simulink model "Biglide_Lee_Palma"  (R2019b)
settings: Solver=VariableStepAuto  StartTime=0.0  StopTime=3  RelTol=1e-3
values from neighbouring files (symbols this model uses):
  ADAMS_communication_interval = 0.005    [Controls_Plant_1.m]    (also in Controls_Plant_3.m; Controls_Plant_5.m)
  ADAMS_communications_per_output_step = 1    [Controls_Plant_1.m]    (also in Controls_Plant_3.m; Controls_Plant_5.m)
  ADAMS_cwd = 'C:\Users\Justin\Documents\EMARO+\Centrale Nantes\Courses\AMORO\Lab\Lab 4'    [Controls_Plant_1.m]    (also in Controls_Plant_3.m; Controls_Plant_5.m)
  ADAMS_exec = ''    [Controls_Plant_1.m]    (also in Controls_Plant_3.m; Controls_Plant_5.m)
  ADAMS_host = 'LAPTOP-CH4PO0JS'    [Controls_Plant_1.m]    (also in Controls_Plant_3.m; Controls_Plant_5.m)
  ADAMS_init = ''    [Controls_Plant_1.m]    (also in Controls_Plant_3.m; Controls_Plant_5.m)
  ADAMS_inputs = 'dummy_input'    [Controls_Plant_1.m]    (also in Controls_Plant_3.m = 'q1d!q2d'; Controls_Plant_5.m = 'f1!f2')
  ADAMS_outputs = 'x!y!xd!yd!xdd!ydd!phi1!phi2!phi1d!phi2d!phi1dd!phi2dd!f1!f2'    [Controls_Plant_1.m]    (also in Controls_Plant_3.m = 'q1!q2'; Controls_Plant_5.m = 'q1!q2')
  ADAMS_prefix = 'Controls_Plant_1'    [Controls_Plant_1.m]    (also in Controls_Plant_3.m = 'Controls_Plant_3'; Controls_Plant_5.m = 'Controls_Plant_5')
  ADAMS_static = 'no'    [Controls_Plant_1.m]    (also in Controls_Plant_3.m; Controls_Plant_5.m)
  ADAMS_sysdir = 'C:\PROGRA~1\MSC~1.SOF\ADAMSS~1\2020_1\'    [Controls_Plant_1.m]    (also in Controls_Plant_3.m; Controls_Plant_5.m)
  ADAMS_time_offset = 0.0    (= 0)    [Controls_Plant_1.m]    (also in Controls_Plant_3.m; Controls_Plant_5.m)
settings Model: Creator=Steven  LastModifiedBy=Justin
settings DataIOCC: ReturnWorkspaceOutputs=off
settings DebuggingCC: ArithmeticOperatorsInVariantConditions=warning
settings SFSimCC: SimUseLocalCustomCode=off  CustomCodeUndefinedFunction=UseInterfaceOnly
settings RTWCC: RTWUseLocalCustomCode=off

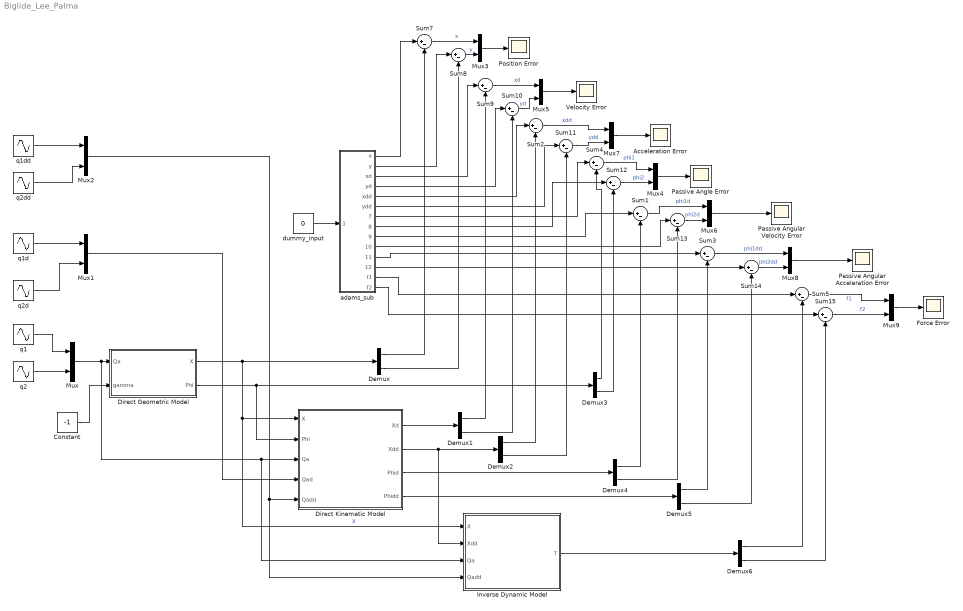
== system Biglide_Lee_Palma ==
  Acceleration Error : Scope
  Constant : Constant  Value=-1
  Demux{,1..6} (7 alike) : Demux  Outputs=2
  Direct Geometric Model : MATLAB Function  TreatAsAtomicUnit=on
  Direct Kinematic Model : MATLAB Function  TreatAsAtomicUnit=on
  Force Error : Scope
  Inverse Dynamic Model : MATLAB Function  TreatAsAtomicUnit=on
  Mux{,1..9} (10 alike) : Mux  Inputs=2
  Passive Angle Error : Scope
  Passive Angular Acceleration Error : Scope
  Passive Angular Velocity Error : Scope
  Position Error : Scope
  Sum{1..5,7..15} (14 alike) : Sum  Inputs=|+-
  Velocity Error : Scope
  adams_sub : Subsystem
  dummy_input : Constant  Value=0
  q1 : Sin  Amplitude=0.1  SampleTime=0
  q1d : Sin  Amplitude=0.1  Phase=+pi/2  SampleTime=0
  q1dd : Sin  Amplitude=0.1  Phase=+pi  SampleTime=0
  q2 : Sin  Amplitude=-0.1  SampleTime=0
  q2d : Sin  Amplitude=-0.1  Phase=pi/2  SampleTime=0
  q2dd : Sin  Amplitude=-0.1  Phase=+pi  SampleTime=0
  wires:
  q1/1 -> Mux/1
  q2/1 -> Mux/2
  Mux/1 -> Inverse Dynamic Model/3(Qa), Direct Kinematic Model/3(Qa), Direct Geometric Model/1(Qa)
  Constant/1 -> Direct Geometric Model/2(gamma)
  Direct Geometric Model/2(Phi) -> Direct Kinematic Model/2(Phi), Demux3/1
  q1d/1 -> Mux1/1
  q2d/1 -> Mux1/2
  Mux1/1 -> Direct Kinematic Model/4(Qad)
  q1dd/1 -> Mux2/1
  q2dd/1 -> Mux2/2
  Mux2/1 -> Inverse Dynamic Model/4(Qadd), Direct Kinematic Model/5(Qadd)
  Direct Kinematic Model/1(Xd) -> Demux1/1
  Direct Kinematic Model/2(Xdd) -> Demux2/1, Inverse Dynamic Model/2(Xdd)
  Direct Kinematic Model/3(Phid) -> Demux4/1
  Direct Kinematic Model/4(Phidd) -> Demux5/1
  adams_sub/14("f2    ") -> Sum15/1
  adams_sub/13("f1    ") -> Sum5/1
  adams_sub/12(phi2dd) -> Sum14/1
  adams_sub/11(phi1dd) -> Sum3/1
  adams_sub/10("phi2d ") -> Sum13/1
  adams_sub/9("phi1d ") -> Sum1/1
  adams_sub/8("phi2  ") -> Sum12/1
  adams_sub/7("phi1  ") -> Sum4/1
  adams_sub/6("ydd   ") -> Sum11/1
  adams_sub/5("xdd   ") -> Sum2/1
  adams_sub/4("yd    ") -> Sum10/1
  adams_sub/3("xd    ") -> Sum9/1
  adams_sub/2("y     ") -> Sum8/1
  adams_sub/1("x     ") -> Sum7/1
  dummy_input/1 -> adams_sub/1(dummy_input)
  Mux3/1 -> Position Error/1
  Mux4/1 -> Passive Angle Error/1
  Mux5/1 -> Velocity Error/1
  Mux7/1 -> Acceleration Error/1
  Mux8/1 -> Passive Angular Acceleration Error/1
  Mux9/1 -> Force Error/1
  Direct Geometric Model/1(X) -> Inverse Dynamic Model/1(X), Direct Kinematic Model/1(X), Demux/1  "X"
  Sum7/1 -> Mux3/1  "x"
  Demux/1 -> Sum7/2
  Demux/2 -> Sum8/2
  Sum8/1 -> Mux3/2  "y"
  Demux1/1 -> Sum9/2
  Demux1/2 -> Sum10/2
  Sum9/1 -> Mux5/1  "xd"
  Sum10/1 -> Mux5/2  "yd"
  Demux2/1 -> Sum2/2
  Demux2/2 -> Sum11/2
  Sum2/1 -> Mux7/1  "xdd"
  Sum11/1 -> Mux7/2  "ydd"
  Sum12/1 -> Mux4/2  "phi2"
  Sum4/1 -> Mux4/1  "phi1"
  Demux3/1 -> Sum4/2
  Demux3/2 -> Sum12/2
  Sum1/1 -> Mux6/1  "phi1d"
  Sum13/1 -> Mux6/2  "phi2d"
  Demux4/1 -> Sum1/2
  Demux4/2 -> Sum13/2
  Mux6/1 -> Passive Angular Velocity Error/1
  Sum14/1 -> Mux8/2  "phi2dd"
  Sum3/1 -> Mux8/1  "phi1dd"
  Demux5/1 -> Sum3/2
  Demux5/2 -> Sum14/2
  Inverse Dynamic Model/1(T) -> Demux6/1
  Sum5/1 -> Mux9/1  "f1"
  Sum15/1 -> Mux9/2  "f2"
  Demux6/1 -> Sum5/2
  Demux6/2 -> Sum15/2

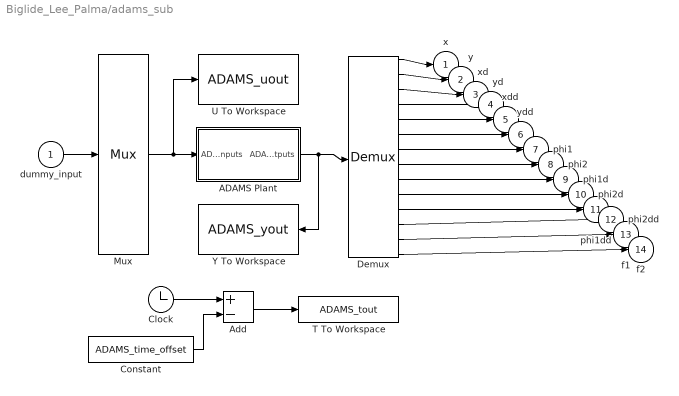
== system Biglide_Lee_Palma/adams_sub ==
  dummy_input : Inport
  ADAMS Plant : Subsystem  LoadFcn=|  InitFcn=clear mex  mask(Adams Plant){exevie=ADAMS_sysdir, nam_in=ADAMS_inputs, namout=ADAMS_outputs, nampre=ADAMS_prefix, outfil=ADAMS_prefix, exesol=ADAMS_exec, stat=ADAMS_static, inicmd=[ADAMS_init], exetyp=C++, comtyp=PIPE(DDE), workdir=ADAMS_cwd, ada_host=ADAMS_host, modani=interactive, modsim=discrete, dft=no, simulink_lead_cosim=yes, pin_interp_order=0, pout_extrap_order=0, pin_extrap_order=0, pout_interp_order=0, dt_out=ADAMS_communication_interval, o_rate=ADAMS_communications_per_output_step, time_offset=ADAMS_time_offset, more=off}
      | %check based on dialog box setting for when setting by popup menu                                             
      | if exist('ADAMS_solver_type')                                                                                 
      |   if strcmp(ADAMS_solver_type,'C++')                                                                          
      |     set_param(gcb,'exetyp','C++');                                                                            
      |   else                                                                                                        
      |     set_param(gcb,'exetyp','Fortran');                                                                        
      |   end                                                                                                         
      | else                                                                                                          
      |   set_param(gcb,'exetyp','C++');                                                                              
      | end                                                                                                           
      | %set the mode if using acar_solver                                                                            
      | %REQUIRED HERE BECAUSE BELOW CAUSES MDLTERMINATE TO BE CALLED 2 TIMES IN MIDDLE OF SIMULATION WHEN SET IN MASK
      |                                                                                                               
      | %enable the direct feedthrough, sim mode, anim mode parameters by default                                     
      |                                                                                                               
      | if exist('set_some_params_states')                                                                            
      |                                                                                                               
      |   set_some_params_states({'dft','modsim','modani'},{'on','on','on'},'MaskEnables',gcb)                        
      |   %turn on direct feedthrough option                                                                          
      |   set_some_params_states({'dft'},{'on'},'MaskVisibilities',gcb)                                               
      |                                                                                                               
      |  end                                                                                                          
      |                                                                                                               
      |                                                                                                               
      | if exist('ADAMS_exec')                                                                                        
      |   if and(strcmp(get_param(gcb,'exesol'),'ADAMS_exec'),strcmp(ADAMS_exec,'acar_solver'))                       
      |     %set the sim mode to discrete -- only supported mode                                                      
      |     set_param(gcb,'modsim','discrete')                                                                        
      |      %turn off direct feedthrough option                                                                      
      |      set_some_params_states({'dft'},{'off'},'MaskVisibilities',gcb)                                           
      |     %set the animation mode to batch -- only supported mode                                                   
      |     set_param(gcb,'modani','batch')                                                                           
      |     %disable the direct feedthrough, sim mode, anim mode parameters                                           
      |     set_some_params_states({'modsim','modani'},{'off','off'},'MaskEnables',gcb)                               
      |   end
      |   if and(strcmp(get_param(gcb,'exesol'),'ADAMS_exec'),strcmp(ADAMS_exec,'apre_solver'))                       
      |     %set the sim mode to discrete -- only supported mode                                                      
      |     set_param(gcb,'modsim','discrete')                                                                        
      |      %turn off direct feedthrough option                                                                      
      |      set_some_params_states({'dft'},{'off'},'MaskVisibilities',gcb)                                           
      |     %set the animation mode to batch -- only supported mode                                                   
      |     set_param(gcb,'modani','batch')                                                                           
      |     %disable the direct feedthrough, sim mode, anim mode parameters                                           
      |     set_some_params_states({'modsim','modani'},{'off','off'},'MaskEnables',gcb)                               
      |   end                                                                                                  
      | end
      mask prompts: exevie "Adams install directory"; nam_in "Adams View input names"; namout "Adams View output names"; nampre "Adams model file prefix"; outfil "Output files prefix (opt.: if blank - no output)"; exesol "User executable (opt.: if blank - use standard)"; stat "Initial static simulation flag"; inicmd "Initialization commands"; exetyp "Adams Solver type"; comtyp "Interprocess option"; workdir "Adams working directory"; ada_host "Adams host"; modani "Animation mode"; modsim "Simulation mode"; dft "Direct feedthrough"; simulink_lead_cosim "Discrete Computational Order - Simulink Leads Adams"; pin_interp_order "Plant input interpolation order"; pout_extrap_order "Plant output extrapolation order"; pin_extrap_order "Plant input extrapolation order"; pout_interp_order "Plant output interpolation order"; dt_out "Communication interval"; o_rate "Number of communications per output step"; time_offset "Offset between Simulink and Adams simulation time"; more "More parameters"
      mask help: Simulate any Adams plant model either in Adams Solver form (.adm file) or in Adams View form (.cmd file)
      settings: OpenFcn=|
      | open_system(gcb,'mask')
      | if not(exist('set_some_params_states'))
      | 
      | warning('The script "set_some_params_states.m" cannot be found in the MATLAB PATH.  Cannot update the ADAMS Plant S-Function parameters.')
      | 
      | warning('Recommended action(optional):  run the Adams Controls .m file first to help choose the correct settings in the Adams S-Function block.')
      | 
      | end
      mask Help:
      | <html>
      | This S-Function represents the non-linear Adams Plant with the inputs sent to the Adams model as input #1 and Time as input #2<br>
      |  and the outputs generated by the Adams model.  See the Adams Controls documentation for more <br>
      | information.  This plant uses the following variables:<br>
      | <br>
      | <b>ADAMS_sysdir:</b> Adams installation directory<br>
      | <b>ADAMS_inputs:</b> Input variables View names vector<br>
      | <b>ADAMS_outputs :</b> Outputs variables View names vector<br>
      | <b>ADAMS_prefix:</b> ADAMS model files prefix (.adm, .cmd); also doubles as output files prefix<br>
      | <b>ADAMS_exec:</b>  Adams Solver user library or keyword (e.g., acar_solver)<br>
      | <b>ADAMS_static:</b> yes|no - initial static before Co-simulation(discrete)/Function Evaluation(continuous)<br>
      | <b>ADAMS_init:</b> Initialization commands (i.e., Adams View or Solver commands, depending on setting for Animation mode)<br>
      | <b>ADAMS_cwd:</b> Current working directory (for TCP/IP)<br>
      | <b>ADAMS_host:</b> Name of Adams server host (for TCP/IP)<br>
      | <b>ADAMS_mode:</b> Linear or non-linear (i.e., co-sim, function eval)<br>
      | <b>ADAMS_solver_type:</b> Fortran or C++ (used to set popup menu when first loaded)<br>
      | <b>ADAMS_communication_interval:</b> Time step at which Co-simulation exchange information (e.g.,0.005); also controls <br>output for continuous mode (Function Evaluation)<br>
      | <b>ADAMS_communications_per_output_step: </b>Sets Adams output rate (.res, .req, .gra) integer value (default: 1)<br>
      | <b>ADAMS_time_offset: </b>Removes this time offset from simulation time used by Adams. Adams will be sent a time value being Simulink simulation time - this value. (default: 0). Eg. if ADAMS_time_offset=2: if Simulink time=2 then Adams time = 0. Make sure that the Adams block is disabled when the Adams time is <0. If not an error will be raised. <br>
      | 
      | 
      | <br>
      | The following settings can be chosen:<br>
      | <br>
      | <b>Adams Solver type:</b>  Fortran or C++ (will also set ADAMS_solver_type)<br>
      | <b>Interprocess option:</b> Pipe(DDE), TCP/IP or DIRECT; TCP/IP can allow different machines run Adams and MATLAB<br>
      | <b>Animation mode:</b> batch (Solver, uses .adm) or interactive (View, uses .cmd)<br>
      | <b>Simulation mode:</b> discrete (Co-simulation) or continuous (Function Evaluation)<br>
      | <b>Discrete Computational Order - Simulink Lead Adams:</b> for discrete mode, chooses if Simulink leads the integration (yes) or lags (no);<br> if set to "no", can remove algebraic loop<br>
      | <b>Plant input interpolation order:</b> 0 = zero-order hold; 1 = linear (discrete mode only, where Simulink leads)<br>
      | <b>Plant output extrapolation order:</b> 0 = zero-order hold;1 = linear(discrete mode only, where Simulink leads)<br>
      | <b>Plant input extrapolation order:</b> 0 = zero-order hold; 1 = linear (discrete mode only, where Adams leads)<br>
      | <b>Plant output interpolation order:</b> 0 = zero-order hold;1 = linear(discrete mode only, where Adams leads)<br>
      | <b>Direct feedthrough:</b> yes|no - yes = Input directly effect output(continuous mode-only)<br>
      | 
      | </html>
      mask Callback exesol:
      | if exist('set_some_params_states')
      | %enable the direct feedthrough, sim mode, anim mode parameters
      | set_some_params_states({'dft','modsim','modani'},{'on','on','on'},'MaskEnables',gcb)
      | %turn on direct feedthrough option
      | set_some_params_states({'dft'},{'on'},'MaskVisibilities',gcb)
      | end
      | 
      | if exist('ADAMS_exec')
      |   if and(strcmp(get_param(gcb,'exesol'),'ADAMS_exec'),strcmp(ADAMS_exec,'acar_solver'))
      |     %set the sim mode to discrete -- only supported mode
      |     %REMOVED:  BELOW CAUSES MDLTERMINATE TO BE CALLED 2 TIMES IN MIDDLE OF SIMULATION
      |     %Now in LoadFcn callback
      |     %set_param(gcb,'modsim','discrete')
      |      %turn off direct feedthrough option
      |     set_some_params_states({'dft'},{'off'},'MaskVisibilities',gcb)
      |     %set the animation mode to batch -- only supported mode
      |     %REMOVED:  BELOW CAUSES MDLTERMINATE TO BE CALLED 2 TIMES IN MIDDLE OF SIMULATION
      |     %Now in LoadFcn callback
      |     %set_param(gcb,'modani','batch')
      |     %disable the direct feedthrough, sim mode, anim mode parameters
      |     set_some_params_states({'modsim','modani'},{'off','off'},'MaskEnables',gcb)
      |   end
      | end
      mask TypeOptions exetyp: Fortran | C++
      mask Callback exetyp:
      | if strcmp(get_param(gcb,'exetyp'),'C++')
      |     ADAMS_solver_type='C++';
      | else
      |     ADAMS_solver_type='Fortran';
      | end
      mask TypeOptions comtyp: PIPE(DDE) | TCP/IP | DIRECT
      mask Callback comtyp:
      | if exist('set_some_params_states')
      | if strcmp(get_param(gcb,'comtyp'),'PIPE(DDE)') || strcmp(get_param(gcb,'comtyp'),'DIRECT')
      |     %turn off cwd, host options
      |     set_some_params_states({'ada_host','workdir'},{'off','off'},'MaskVisibilities',gcb)
      | else%if strcmp(get_param(gcb,'modsim'),'TCP/IP')
      |     %turn on cwd, host options
      |     set_some_params_states({'ada_host','workdir'},{'on','on'},'MaskVisibilities',gcb)
      | end
      | end
      mask TypeOptions modani: batch | interactive
      mask TypeOptions modsim: discrete | continuous
      mask Callback modsim:
      | if exist('set_some_params_states')
      | if strcmp(get_param(gcb,'modsim'),'discrete')
      |      %turn off direct feedthrough option
      |     set_some_params_states({'dft'},{'off'},'MaskVisibilities',gcb)
      |     %turn on discrete co-sim type if want to see more
      |     if strcmp(get_param(gcb,'more'),'on')
      |         set_some_params_states({'simulink_lead_cosim'},{'on'},'MaskVisibilities',gcb)
      |     end
      |     if strcmp(get_param(gcb,'simulink_lead_cosim'),'yes')
      |         %turn on interpolation/extrapolation options
      |         set_some_params_states({'pin_interp_order','pout_extrap_order',},{'on','on'},'MaskVisibilities',gcb)
      |     else
      |         set_some_params_states({'pin_extrap_order','pout_interp_order'},{'on','on'},'MaskVisibilities',gcb)
      |     end
      | else%if strcmp(get_param(gcb,'modsim'),'continuous')
      |      %turn off direct feedthrough option
      |     set_some_params_states({'dft'},{'on'},'MaskVisibilities',gcb)
      |     %turn off interpolation/extrapolation options
      |     set_some_params_states({'pin_interp_order','pout_extrap_order','pin_extrap_order','pout_interp_order','simulink_lead_cosim'},{'off','off','off','off','off'},'MaskVisibilities',gcb)
      | end
      | end
      mask TypeOptions dft: no | yes
      mask TypeOptions simulink_lead_cosim: yes | no
      mask Callback simulink_lead_cosim:
      | if exist('set_some_params_states')
      | if (strcmp(get_param(gcb,'simulink_lead_cosim'),'yes') && strcmp(get_param(gcb,'modsim'),'discrete'))
      |      %turn off unused interpolate/extrapolate options
      |     set_some_params_states({'pin_extrap_order','pout_interp_order'},{'off','off'},'MaskVisibilities',gcb)
      |     %turn on used interpolate/extrapolate options
      |     set_some_params_states({'pin_interp_order','pout_extrap_order'},{'on','on'},'MaskVisibilities',gcb)
      | elseif (strcmp(get_param(gcb,'simulink_lead_cosim'),'no') && strcmp(get_param(gcb,'modsim'),'discrete'))
      |     %turn on used interpolate/extrapolate options
      |     set_some_params_states({'pin_extrap_order','pout_interp_order'},{'on','on'},'MaskVisibilities',gcb)
      |      %turn off unused interpolate/extrapolate options
      |     set_some_params_states({'pin_interp_order','pout_extrap_order'},{'off','off'},'MaskVisibilities',gcb)
      | end
      | end
      mask TypeOptions pin_interp_order: 0 | 1
      mask TypeOptions pout_extrap_order: 0 | 1
      mask TypeOptions pin_extrap_order: 0 | 1
      mask TypeOptions pout_interp_order: 0 | 1
      mask Callback more:
      | if exist('set_some_params_states')
      | if (strcmp(get_param(gcb,'more'),'on'))
      |      %turn on infrequently used options
      |     set_some_params_states({'exevie','nam_in','namout','exesol','stat','inicmd','time_offset'},{'on','on','on','on','on','on','on'},'MaskVisibilities',gcb)
      |     if strcmp(get_param(gcb,'modsim'),'discrete')
      |         set_some_params_states({'simulink_lead_cosim'},{'on'},'MaskVisibilities',gcb)
      |     end
      | elseif (strcmp(get_param(gcb,'more'),'off'))
      |     %turn off infrequently used options
      |     set_some_params_states({'exevie','nam_in','namout','exesol','stat','inicmd','time_offset'},{'off','off','off','off','off','off','off'},'MaskVisibilities',gcb)
      |     if strcmp(get_param(gcb,'modsim'),'discrete')
      |         set_some_params_states({'simulink_lead_cosim'},{'off'},'MaskVisibilities',gcb)
      |     end
      | end
      | end
      mask Display: disp( 'MSC Software' )
  Add : Sum  Inputs=+-
  Clock : Clock
  Constant : Constant  Value=ADAMS_time_offset
  Demux : Demux  Outputs=14
  Mux : Mux  Inputs=1
  T To Workspace : ToWorkspace  VariableName=ADAMS_tout
      settings: MaxDataPoints=100000
  U To Workspace : ToWorkspace  VariableName=ADAMS_uout
      settings: MaxDataPoints=100000
  Y To Workspace : ToWorkspace  VariableName=ADAMS_yout
      settings: MaxDataPoints=100000
  "x     " : Outport
  "y     " : Outport  Port=2
  "xd    " : Outport  Port=3
  "yd    " : Outport  Port=4
  "xdd   " : Outport  Port=5
  "ydd   " : Outport  Port=6
  "phi1  " : Outport  Port=7
  "phi2  " : Outport  Port=8
  "phi1d " : Outport  Port=9
  "phi2d " : Outport  Port=10
  phi1dd : Outport  Port=11
  phi2dd : Outport  Port=12
  "f1    " : Outport  Port=13
  "f2    " : Outport  Port=14
  wires:
  Mux/1 -> ADAMS Plant/1(ADAMS inputs), U To Workspace/1
  ADAMS Plant/1(ADAMS outputs) -> Demux/1, Y To Workspace/1
  Clock/1 -> Add/1
  Constant/1 -> Add/2
  Add/1 -> T To Workspace/1
  Demux/1 -> "x     "/1
  Demux/2 -> "y     "/1
  Demux/3 -> "xd    "/1
  Demux/4 -> "yd    "/1
  Demux/5 -> "xdd   "/1
  Demux/6 -> "ydd   "/1
  Demux/7 -> "phi1  "/1
  Demux/8 -> "phi2  "/1
  Demux/9 -> "phi1d "/1
  Demux/10 -> "phi2d "/1
  Demux/11 -> phi1dd/1
  Demux/12 -> phi2dd/1
  Demux/13 -> "f1    "/1
  Demux/14 -> "f2    "/1
  dummy_input/1 -> Mux/1

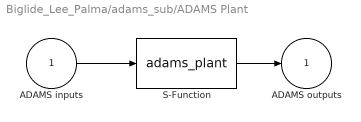
== system Biglide_Lee_Palma/adams_sub/ADAMS Plant ==
  ADAMS inputs : Inport
  S-Function : S-Function  StopFcn=clear mex  FunctionName=adams_plant  Parameters=exevie,exesol,stat,outfil,nampre,o_rate,nam_in,namout,dft,modsim,modani,dt_out,inicmd,exetyp,comtyp,ada_host, workdir,pin_interp_order,pout_extrap_order,pin_extrap_order,pout_interp_order,simulink_lead_cosim,time_offset  SFunctionDeploymentMode=off  EnableBusSupport=off
  ADAMS outputs : Outport  InitialOutput=0
  wires:
  ADAMS inputs/1 -> S-Function/1
  S-Function/1 -> ADAMS outputs/1

== matlab function Biglide_Lee_Palma/Direct Kinematic Model ==
  data: X input; Phi input; Xd output; Qa input; Qad input; Xdd output; Qadd input; Phid output; Phidd output
function [Xd, Xdd, Phid, Phidd]  = DKM(X,Phi,Qa,Qad,Qadd)
    
    %% Geometric parameters
    d= 0.4;
    l= 0.3606;
    
    % Extracting Parameters
    x = X(1);
    y = X(2);
    phi1 = Phi(1);
    phi2 = Phi(2);
    q1 = Qa(1);
    q2 = Qa(2);
    q1d = Qad(1);
    q2d = Qad(2);
    
    %% First derivative of X (Xd)
    A = 2*[(x+d/2) (y-q1); (x-d/2) (y-q2)];
    B = -2*[(y-q1) 0; 0 (y-q2)];
    
    Xd = -A\(B*Qad);
    
    xd = Xd(1);
    yd = Xd(2);
    
    %% Second derivative of X (Xdd)
    Ad= 2*[(xd) (yd-q1d); (xd) (yd-q2d)];
    Bd= -2*[(yd-q1d) 0; 0 (yd-q2d)];
    
    Xdd= -A\(B*Qadd + Ad*Xd + Bd*Qad);
    
    %% First derivative of the Passive Angles (Phid)
    Aq = l*[-sin(phi1) sin(phi2); cos(phi1) -cos(phi2)];
    Bq = [0 0; 1 -1];
    
    Phid = -Aq\(Bq*Qad);
    
    phi1d = Phid(1);
    phi2d = Phid(2);
    
    %% Second derivative of the Passive Angles (Phidd)
    Aqd= l*[-cos(phi1)*phi1d cos(phi2)*phi2d; -sin(phi1)*phi1d sin(phi2)*phi2d];
    Bqd=[0 0; 0 0];
    
    Phidd=-Aq\(Bq*Qadd + Aqd*Phid + Bqd*Qad);  
end

== matlab function Biglide_Lee_Palma/Direct Geometric Model ==
  data: Qa input; X output; gamma input; Phi output
function [X, Phi] = DGM(Qa,gamma)
    
    % Geometric parameters
    d = 0.4;
    l = 0.3606;
    
    q1 = Qa(1);
    q2 = Qa(2);
    
    % Segments
    OA = [d/2; q2];
    AM = [-d; q1-q2]/2;
    MC = gamma * sqrt((4*l^2 - d^2 -(q1-q2)^2)/(d^2 + (q1-q2)^2)) * [0 -1; 1 0] * AM;
    
    X= OA + AM + MC;
    
    x=X(1);
    y=X(2);
    
    % Passive Angles
    Phi= [atan2(y-q1,x+d/2); atan2(y-q2,x-d/2)];
end

== matlab function Biglide_Lee_Palma/Inverse Dynamic Model ==
  data: X input; Xdd input; T output; Qa input; Qadd input
function T = IDM(X, Xdd, Qa, Qadd)

%% Geometric and Dynamic variables
d = 0.4;
mp = 3;
mf = 1;

%Extracting variables from inputs
q1 = Qa(1);
q2 = Qa(2);
q1dd = Qadd(1);
q2dd = Qadd(2);
x = X(1);
y = X(2);
xdd = Xdd(1);
ydd = Xdd(2);

%% Calculating the Jacobian
A = 2*[(x + d/2) (y - q1) ; (x - d/2) (y - q2)];
B = -2*[(y - q1) 0 ; 0 (y-q2)]; 

J = -A\B;

%% Calculate Torque based off equation T = M + c
M = mf*[q1dd ; q2dd];
c = J'*mp*[xdd ; ydd];

T = M + c;
end
